simulink model "gm_sampleModel1976_sub"  (R2023a)
settings: Solver=VariableStepAuto  StartTime=0.0  StopTime=10.0  RelTol=1e-3
libraries: simulink x1, hdlsllib x1
settings Model: Creator=user1  LastModifiedBy=user1
settings OptimizationCC: BlockReduction=off  ConditionallyExecuteInputs=off
settings DebuggingCC: InheritedTsInSrcMsg=none

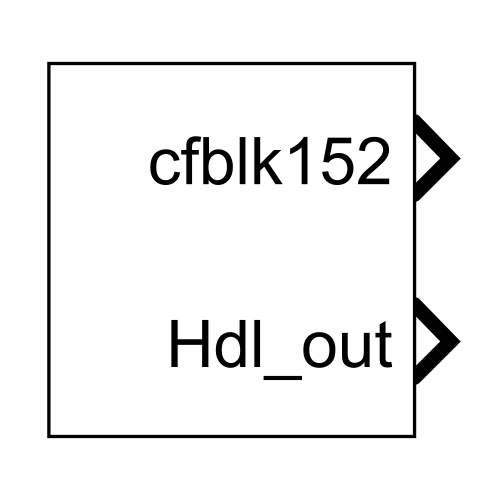
[thumbnail: Simulink's stored preview of the top-level diagram]
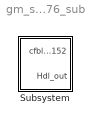
== system gm_sampleModel1976_sub ==
  Subsystem : Subsystem

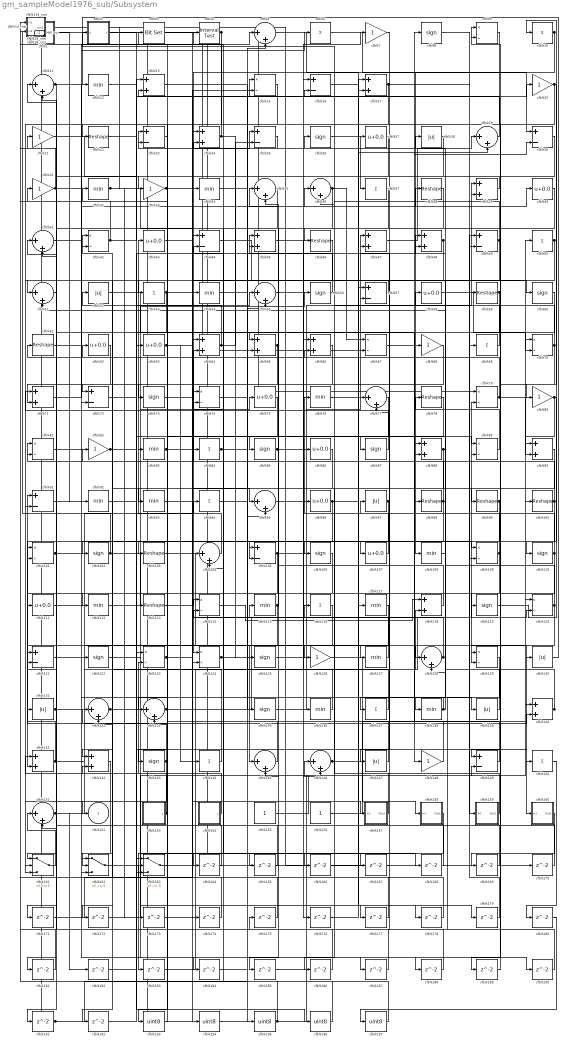
== system gm_sampleModel1976_sub/Subsystem ==
  cfblk1 : Subsystem  mask(Compare To Constant){relop=<=, const=double(3), OutDataTypeStr=uint8, ZeroCross=on}
      mask prompts: relop "Simulink:masks:Operator_MP"; const "Simulink:masks:ConstantValue_MP"; OutDataTypeStr "Simulink:masks:OutputDataType_MP"; ZeroCross "Simulink:masks:EnableZerocrossingDetection_MP"
      mask help: Simulink:masks:CompareToConstant_MD
      mask init:
      | OutDataTypeStr = 'uint8';
      | ZeroCross = 'on';
      | blkName = 'sampleModel1976_sub/Subsystem/cfblk1';
      | const = double(3);
      | const_str = '3.0';
      | const_val = double(3);
      | relop = '<=';
      | setValue = 'fixdt(0, 8)';
      | str = '<= 3';
      mask TypeOptions relop: == | ~= | < | <= | >= | >
      mask TypeOptions OutDataTypeStr: Simulink:masks:uint8 | Simulink:masks:boolean
      mask Callback ZeroCross: sl('zeroCrossEnable', gcbh);
      mask Display: disp(str)
  cfblk{6,10,37,50,53,69,84,94,116,137,144,150} (12 alike) : Sum  Inputs=+  OutDataTypeStr=uint8
  cfblk{22,38,46,59,61,78,98..100,103,113} (11 alike) : Reshape
  cfblk{9,15,42,67,70,74,79,81,89,101,109,114,120,123..124,129} (16 alike) : Product  Inputs=*/  OutDataTypeStr=uint8  RndMeth=Zero  SaturateOnIntegerOverflow=on
  cfblk{8,26,56,60,73,85,87,102,106,110,119,122,125,135,143} (15 alike) : Signum
  cfblk{5,11,29,35..36,41,51,55,77,95,104,128,132..133,145..146,151} (17 alike) : Sum  Inputs=|++  OutDataTypeStr=uint8
  cfblk{16,23,25,30,44,49,57,72,91,105,121,149} (12 alike) : Sum  Inputs=+-  OutDataTypeStr=uint8
  cfblk{27,40,43,58,62..63,75,86,96,107,111} (11 alike) : Bias  Bias=0.0  SaturateOnIntegerOverflow=off
  cfblk{12,32,34,54,76,83,92..93,108,112,115,117,127,136,138} (15 alike) : MinMax  OutDataTypeStr=uint8
  cfblk{13,17,24,39,45,47..48,64..66,71,88,90,118,140..142} (17 alike) : Sum  OutDataTypeStr=uint8
  cfblk{7,20..21,31,33,68,80,82,126,148} (10 alike) : Gain  OutDataTypeStr=uint8
  cfblk{28,52,97,130..131,139,147} (7 alike) : Abs  OutDataTypeStr=uint8  SaturateOnIntegerOverflow=off
  cfblk134_inst : Subsystem
  cfblk14_inst : Subsystem
  cfblk153 : Subsystem  mask(Counter Limited){uplimit=double(7), tsamp=double(-1)}
      mask prompts: uplimit "Simulink:masks:UpperLimit_MP"; tsamp "Simulink:masks:SampleTime_MP"
      mask help: Simulink:masks:CounterLimited_MD
      mask init:
      | nbits = double(8);
      | tsamp = double(-1);
      | uplimit = double(7);
  cfblk154 : Subsystem  mask(Counter Limited){uplimit=double(7), tsamp=double(-1)}
      mask prompts: uplimit "Simulink:masks:UpperLimit_MP"; tsamp "Simulink:masks:SampleTime_MP"
      mask help: Simulink:masks:CounterLimited_MD
      mask init:
      | nbits = double(8);
      | tsamp = double(-1);
      | uplimit = double(7);
  cfblk155 : Constant  OutDataTypeStr=uint8  SampleTime=-1
  cfblk156 : Constant  OutDataTypeStr=uint8  SampleTime=-1
  cfblk157 : Subsystem
  cfblk158 : Subsystem
  cfblk159 : Subsystem
  cfblk160 : Subsystem
  cfblk161 : Switch  OutDataTypeStr=uint8  SaturateOnIntegerOverflow=off  InputSameDT=off
  cfblk162 : Switch  OutDataTypeStr=uint8  SaturateOnIntegerOverflow=off  InputSameDT=off
  cfblk163 : Switch  OutDataTypeStr=uint8  SaturateOnIntegerOverflow=off  InputSameDT=off
  cfblk{164..192} (29 alike) : Delay  SampleTime=1
  cfblk18_inst : Subsystem
  cfblk{193..197} (5 alike) : DataTypeConversion  OutDataTypeStr=uint8  SaturateOnIntegerOverflow=off  RndMeth=Floor
  cfblk19_inst : Subsystem
  cfblk2 : Subsystem  mask(Detect Rise Nonnegative){vinit=double(0), InputProcessing=Elements as channels (sample based), OutDataTypeStr=uint8}
      mask prompts: vinit "Simulink:masks:InitialCondition_MP"; InputProcessing "Simulink:masks:InputProcessing_MP"; OutDataTypeStr "Simulink:masks:OutputDataType_MP"
      mask help: Simulink:masks:DetectRiseNonnegative_MD
      mask init:
      | InputProcessing = 'Elements as channels (sample based)';
      | OutDataTypeStr = 'uint8';
      | vinit = double(0);
      mask TypeOptions InputProcessing: Simulink:masks:ColumnsAsChannelsFrameBased | Simulink:masks:ElementsAsChannelsSampleBased
      mask TypeOptions OutDataTypeStr: Simulink:masks:uint8 | Simulink:masks:boolean
      mask Display: fprintf('U >= 0\n&  NOT\nU/z >= 0')
  cfblk3 : simulink/Logic and Bit Operations/Bit Set  iBit=0
      settings: LibrarySourceBlock=|
      | hdlsllib/Logic and Bit
      | Operations/Bit Set
  cfblk4 : hdlsllib/Logic and Bit Operations/Interval Test  IntervalClosedRight=on  uplimit=0.5  IntervalClosedLeft=on  lowlimit=-0.5  OutDataTypeStr=uint8
  cfblk152 : Outport  OutDataTypeStr=uint8  SampleTime=1  VectorParamsAs1DForOutWhenUnconnected=off
  Hdl_out : Outport  Port=2  OutDataTypeStr=uint8  SampleTime=1
  wires:
  cfblk1/1(y) -> cfblk92/1
  cfblk10/1 -> cfblk124/1, cfblk108/1
  cfblk100/1 -> cfblk64/2, cfblk141/2, cfblk79/2
  cfblk101/1 -> cfblk118/2, cfblk94/1, cfblk54/1
  cfblk102/1 -> cfblk56/1, cfblk19_inst/2(in2), cfblk177/1
  cfblk103/1 -> cfblk160/1(In1)
  cfblk104/1 -> cfblk43/1
  cfblk105/1 -> cfblk47/1, cfblk39/1, cfblk151/2
  cfblk106/1 -> cfblk115/1
  cfblk107/1 -> cfblk97/1
  cfblk108/1 -> cfblk138/1
  cfblk109/1 -> cfblk129/2, cfblk76/1
  cfblk11/1 -> cfblk122/1, cfblk191/1
  cfblk110/1 -> cfblk161/1, cfblk9/1
  cfblk111/1 -> cfblk145/1
  cfblk112/1 -> cfblk75/1
  cfblk113/1 -> cfblk114/1
  cfblk114/1 -> cfblk118/1
  cfblk115/1 -> cfblk35/2, cfblk124/2
  cfblk116/1 -> cfblk181/1
  cfblk117/1 -> cfblk162/2
  cfblk118/1 -> cfblk35/1
  cfblk119/1 -> cfblk10/1
  cfblk12/1 -> cfblk113/1
  cfblk120/1 -> cfblk58/1, cfblk149/1
  cfblk121/1 -> cfblk188/1
  cfblk122/1 -> cfblk190/1
  cfblk123/1 -> cfblk25/1, cfblk120/2
  cfblk124/1 -> cfblk130/1, cfblk89/2
  cfblk125/1 -> cfblk57/2
  cfblk126/1 -> cfblk158/1(In1)
  cfblk127/1 -> cfblk66/2
  cfblk128/1 -> cfblk114/2, cfblk116/1
  cfblk129/1 -> cfblk175/1
  cfblk13/1 -> cfblk55/2
  cfblk130/1 -> cfblk12/1
  cfblk131/1 -> cfblk88/2, cfblk66/1, cfblk16/1
  cfblk132/1 -> cfblk42/1, cfblk168/1
  cfblk133/1 -> cfblk49/2, cfblk68/1
  cfblk134_inst/1(out1) -> cfblk79/1, cfblk170/1
  cfblk135/1 -> cfblk17/2
  cfblk136/1 -> cfblk44/2
  cfblk137/1 -> cfblk74/2
  cfblk138/1 -> cfblk28/1, cfblk137/1
  cfblk139/1 -> cfblk23/1
  cfblk14_inst/1(out1) -> cfblk195/1
  cfblk140/1 -> cfblk62/1, cfblk51/2
  cfblk141/1 -> cfblk91/1, cfblk86/1, cfblk140/2
  cfblk142/1 -> cfblk162/3
  cfblk143/1 -> cfblk23/2, cfblk161/2, cfblk131/1
  cfblk144/1 -> cfblk82/1
  cfblk145/1 -> cfblk61/1
  cfblk146/1 -> cfblk140/1, cfblk120/1
  cfblk147/1 -> cfblk32/1
  cfblk148/1 -> cfblk31/1
  cfblk149/1 -> cfblk81/1
  cfblk15/1 -> cfblk103/1
  cfblk150/1 -> cfblk180/1
  cfblk151/1 -> cfblk8/1, cfblk182/1, cfblk50/1
  cfblk153/1(y) -> cfblk142/2, cfblk141/1, cfblk123/2
  cfblk154/1(y) -> cfblk121/2
  cfblk155/1 -> cfblk70/1
  cfblk156/1 -> cfblk98/1
  cfblk157/1(Out1) -> cfblk2/1(U)
  cfblk158/1(Out1) -> cfblk183/1
  cfblk159/1(Out1) -> cfblk83/1
  cfblk16/1 -> cfblk117/1
  cfblk160/1(Out1) -> cfblk169/1
  cfblk161/1 -> cfblk151/1
  cfblk162/1 -> cfblk167/1
  cfblk163/1 -> cfblk24/1
  cfblk164/1 -> cfblk41/1
  cfblk165/1 -> cfblk64/1
  cfblk166/1 -> cfblk29/2
  cfblk167/1 -> cfblk1/1(u)
  cfblk168/1 -> cfblk13/2
  cfblk169/1 -> cfblk17/1
  cfblk17/1 -> cfblk133/2, cfblk101/2, cfblk159/1(In1)
  cfblk170/1 -> cfblk44/1
  cfblk171/1 -> cfblk74/1
  cfblk172/1 -> cfblk149/2
  cfblk173/1 -> cfblk5/2
  cfblk174/1 -> cfblk42/2
  cfblk175/1 -> cfblk163/2
  cfblk176/1 -> cfblk77/1
  cfblk177/1 -> cfblk132/1
  cfblk178/1 -> cfblk134_inst/1(in1)
  cfblk179/1 -> cfblk49/1
  cfblk18_inst/1(out1) -> cfblk67/2
  cfblk180/1 -> cfblk197/1
  cfblk181/1 -> cfblk19_inst/1(in1)
  cfblk182/1 -> cfblk55/1
  cfblk183/1 -> cfblk146/1
  cfblk184/1 -> cfblk65/2
  cfblk185/1 -> cfblk57/1
  cfblk186/1 -> cfblk81/2
  cfblk187/1 -> cfblk163/1
  cfblk188/1 -> cfblk47/2
  cfblk189/1 -> cfblk9/2
  cfblk19_inst/1(out1) -> cfblk34/1
  cfblk190/1 -> cfblk11/2
  cfblk191/1 -> cfblk95/2, Hdl_out/1
  cfblk192/1 -> cfblk63/1
  cfblk193/1 -> cfblk3/1
  cfblk194/1 -> cfblk119/1
  cfblk195/1 -> cfblk104/2, cfblk100/1
  cfblk196/1 -> cfblk14_inst/1(in1)
  cfblk197/1 -> cfblk14_inst/2(in2)
  cfblk2/1(Y) -> cfblk88/1
  cfblk20/1 -> cfblk80/1, cfblk129/1
  cfblk21/1 -> cfblk123/1
  cfblk22/1 -> cfblk65/1
  cfblk23/1 -> cfblk73/1
  cfblk24/1 -> cfblk18_inst/1(in1), cfblk125/1
  cfblk25/1 -> cfblk24/2
  cfblk26/1 -> cfblk37/1
  cfblk27/1 -> cfblk41/2
  cfblk28/1 -> cfblk121/1
  cfblk29/1 -> cfblk13/1
  cfblk3/1 -> cfblk194/1
  cfblk30/1 -> cfblk99/1
  cfblk31/1 -> cfblk5/1, cfblk18_inst/2(in2), cfblk106/1, cfblk105/2
  cfblk32/1 -> cfblk174/1, cfblk173/1
  cfblk33/1 -> cfblk87/1, cfblk187/1
  cfblk34/1 -> cfblk89/1
  cfblk35/1 -> cfblk104/1
  cfblk36/1 -> cfblk145/2, cfblk67/1
  cfblk37/1 -> cfblk101/1
  cfblk38/1 -> cfblk51/1
  cfblk39/1 -> cfblk33/1
  cfblk4/1 -> cfblk91/2, cfblk171/1
  cfblk40/1 -> cfblk46/1
  cfblk41/1 -> cfblk40/1
  cfblk42/1 -> cfblk134_inst/2(in2), cfblk15/1
  cfblk43/1 -> cfblk60/1
  cfblk44/1 -> cfblk146/2
  cfblk45/1 -> cfblk176/1
  cfblk46/1 -> cfblk84/1
  cfblk47/1 -> cfblk29/1
  cfblk48/1 -> cfblk162/1, cfblk161/3, cfblk132/2
  cfblk49/1 -> cfblk85/1, cfblk16/2
  cfblk5/1 -> cfblk27/1
  cfblk50/1 -> cfblk128/2, cfblk185/1
  cfblk51/1 -> cfblk11/1
  cfblk52/1 -> cfblk148/1
  cfblk53/1 -> cfblk95/1, cfblk71/2
  cfblk54/1 -> cfblk36/1
  cfblk55/1 -> cfblk136/1
  cfblk56/1 -> cfblk45/1
  cfblk57/1 -> cfblk53/1
  cfblk58/1 -> cfblk70/2
  cfblk59/1 -> cfblk147/1, cfblk172/1
  cfblk6/1 -> cfblk30/1
  cfblk60/1 -> cfblk72/1
  cfblk61/1 -> cfblk184/1
  cfblk62/1 -> cfblk111/1
  cfblk63/1 -> cfblk15/2, cfblk144/1
  cfblk64/1 -> cfblk52/1, cfblk25/2
  cfblk65/1 -> cfblk163/3, cfblk112/1
  cfblk66/1 -> cfblk105/1
  cfblk67/1 -> cfblk30/2
  cfblk68/1 -> cfblk72/2
  cfblk69/1 -> cfblk26/1
  cfblk7/1 -> cfblk127/1
  cfblk70/1 -> cfblk36/2, cfblk189/1
  cfblk71/1 -> cfblk6/1
  cfblk72/1 -> cfblk150/1
  cfblk73/1 -> cfblk109/1
  cfblk74/1 -> cfblk135/1
  cfblk75/1 -> cfblk164/1
  cfblk76/1 -> cfblk59/1
  cfblk77/1 -> cfblk193/1
  cfblk78/1 -> cfblk133/1
  cfblk79/1 -> cfblk90/1, cfblk4/1
  cfblk8/1 -> cfblk69/1
  cfblk80/1 -> cfblk90/2, cfblk110/1
  cfblk81/1 -> cfblk107/1
  cfblk82/1 -> cfblk45/2, cfblk192/1
  cfblk83/1 -> cfblk39/2, cfblk157/1(In1)
  cfblk84/1 -> cfblk38/1, cfblk20/1
  cfblk85/1 -> cfblk96/1, cfblk178/1, cfblk109/2
  cfblk86/1 -> cfblk93/1
  cfblk87/1 -> cfblk71/1
  cfblk88/1 -> cfblk48/1, cfblk186/1
  cfblk89/1 -> cfblk78/1
  cfblk9/1 -> cfblk22/1
  cfblk90/1 -> cfblk102/1
  cfblk91/1 -> cfblk139/1
  cfblk92/1 -> cfblk196/1
  cfblk93/1 -> cfblk48/2
  cfblk94/1 -> cfblk126/1
  cfblk95/1 -> cfblk7/1
  cfblk96/1 -> cfblk142/1, cfblk128/1, cfblk179/1
  cfblk97/1 -> cfblk77/2, cfblk166/1
  cfblk98/1 -> cfblk143/1, cfblk21/1
  cfblk99/1 -> cfblk165/1, cfblk152/1

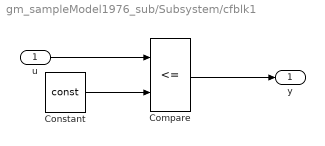
== system gm_sampleModel1976_sub/Subsystem/cfblk1 ==
  u : Inport  OutDataTypeStr=uint8  SampleTime=1
  Compare : RelationalOperator  Operator=<=  OutDataTypeStr=fixdt(0, 8)
  Constant : Constant  DisableCoverage=on  Value=const  OutDataTypeStr=Inherit: Inherit via back propagation  SampleTime=-1
  y : Outport  SampleTime=1
  wires:
  u/1 -> Compare/1
  Compare/1 -> y/1
  Constant/1 -> Compare/2

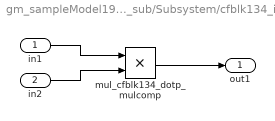
== system gm_sampleModel1976_sub/Subsystem/cfblk134_inst ==
  in1 : Inport  OutDataTypeStr=uint8  SampleTime=1
  in2 : Inport  Port=2  OutDataTypeStr=uint8  SampleTime=1
  mul_cfblk134_dotp_mulcomp : Product  Inputs=**  OutDataTypeStr=uint8  SampleTime=1
  out1 : Outport  OutDataTypeStr=uint8  SampleTime=1
  wires:
  in1/1 -> mul_cfblk134_dotp_mulcomp/1
  in2/1 -> mul_cfblk134_dotp_mulcomp/2
  mul_cfblk134_dotp_mulcomp/1 -> out1/1

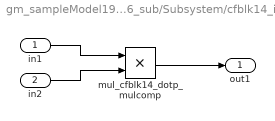
== system gm_sampleModel1976_sub/Subsystem/cfblk14_inst ==
  in1 : Inport  OutDataTypeStr=uint8  SampleTime=1
  in2 : Inport  Port=2  OutDataTypeStr=uint8  SampleTime=1
  mul_cfblk14_dotp_mulcomp : Product  Inputs=**  OutDataTypeStr=uint8  SampleTime=1
  out1 : Outport  OutDataTypeStr=uint8  SampleTime=1
  wires:
  in1/1 -> mul_cfblk14_dotp_mulcomp/1
  in2/1 -> mul_cfblk14_dotp_mulcomp/2
  mul_cfblk14_dotp_mulcomp/1 -> out1/1

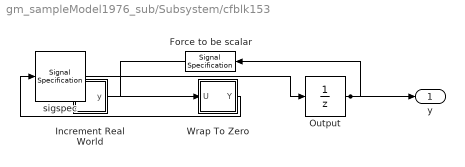
== system gm_sampleModel1976_sub/Subsystem/cfblk153 ==
  Force to be scalar : SignalSpecification  DisableCoverage=on  Dimensions=1
  Increment Real World : Subsystem  mask(Real World Value Increment){}
      mask help: Simulink:masks:RealWorldValueIncrement_MD
      mask Display: disp('V++')
  Output : UnitDelay  InitialCondition=0.0  SampleTime=tsamp  HasFrameUpgradeWarning=on
  Wrap To Zero : Subsystem  mask(Wrap To Zero){Threshold=double(7)}
      mask prompts: Threshold "Simulink:masks:Threshold_MP"
      mask help: Simulink:masks:WrapToZero_MD
  sigspec : SignalSpecification  OutDataTypeStr=uint8  Dimensions=1
  y : Outport  SampleTime=1
  wires:
  Force to be scalar/1 -> Increment Real World/1(u)
  Increment Real World/1(y) -> Wrap To Zero/1(U)
  Output/1 -> Force to be scalar/1, y/1
  Wrap To Zero/1(Y) -> sigspec/1
  sigspec/1 -> Output/1

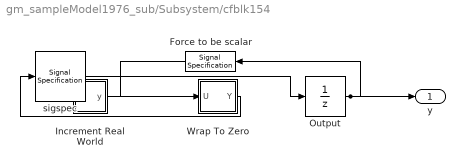
== system gm_sampleModel1976_sub/Subsystem/cfblk154 ==
  Force to be scalar : SignalSpecification  DisableCoverage=on  Dimensions=1
  Increment Real World : Subsystem  mask(Real World Value Increment){}
      mask help: Simulink:masks:RealWorldValueIncrement_MD
      mask Display: disp('V++')
  Output : UnitDelay  InitialCondition=0.0  SampleTime=tsamp  HasFrameUpgradeWarning=on
  Wrap To Zero : Subsystem  mask(Wrap To Zero){Threshold=double(7)}
      mask prompts: Threshold "Simulink:masks:Threshold_MP"
      mask help: Simulink:masks:WrapToZero_MD
  sigspec : SignalSpecification  OutDataTypeStr=uint8  Dimensions=1
  y : Outport  SampleTime=1
  wires:
  Force to be scalar/1 -> Increment Real World/1(u)
  Increment Real World/1(y) -> Wrap To Zero/1(U)
  Output/1 -> Force to be scalar/1, y/1
  Wrap To Zero/1(Y) -> sigspec/1
  sigspec/1 -> Output/1

== system gm_sampleModel1976_sub/Subsystem/cfblk157 ==
  In1 : Inport  OutDataTypeStr=uint8  PortDimensions=1  SampleTime=1
  Out1 : Outport  SampleTime=1
  wires:
  In1/1 -> Out1/1

== system gm_sampleModel1976_sub/Subsystem/cfblk158 ==
  In1 : Inport  OutDataTypeStr=uint8  PortDimensions=1  SampleTime=1
  Out1 : Outport  SampleTime=1
  wires:
  In1/1 -> Out1/1

== system gm_sampleModel1976_sub/Subsystem/cfblk159 ==
  In1 : Inport  OutDataTypeStr=uint8  PortDimensions=1  SampleTime=1
  Out1 : Outport  SampleTime=1
  wires:
  In1/1 -> Out1/1

== system gm_sampleModel1976_sub/Subsystem/cfblk160 ==
  In1 : Inport  OutDataTypeStr=uint8  PortDimensions=1  SampleTime=1
  Out1 : Outport  SampleTime=1
  wires:
  In1/1 -> Out1/1

== system gm_sampleModel1976_sub/Subsystem/cfblk18_inst ==
  in1 : Inport  OutDataTypeStr=uint8  SampleTime=1
  in2 : Inport  Port=2  OutDataTypeStr=uint8  SampleTime=1
  mul_cfblk18_dotp_mulcomp : Product  Inputs=**  OutDataTypeStr=uint8  SampleTime=1
  out1 : Outport  OutDataTypeStr=uint8  SampleTime=1
  wires:
  in1/1 -> mul_cfblk18_dotp_mulcomp/1
  in2/1 -> mul_cfblk18_dotp_mulcomp/2
  mul_cfblk18_dotp_mulcomp/1 -> out1/1

== system gm_sampleModel1976_sub/Subsystem/cfblk19_inst ==
  in1 : Inport  OutDataTypeStr=uint8  SampleTime=1
  in2 : Inport  Port=2  OutDataTypeStr=uint8  SampleTime=1
  mul_cfblk19_dotp_mulcomp : Product  Inputs=**  OutDataTypeStr=uint8  SampleTime=1
  out1 : Outport  OutDataTypeStr=uint8  SampleTime=1
  wires:
  in1/1 -> mul_cfblk19_dotp_mulcomp/1
  in2/1 -> mul_cfblk19_dotp_mulcomp/2
  mul_cfblk19_dotp_mulcomp/1 -> out1/1

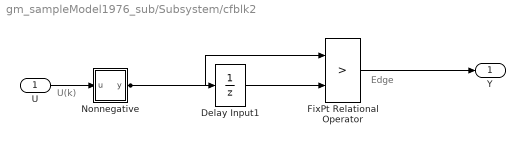
== system gm_sampleModel1976_sub/Subsystem/cfblk2 ==
  note: U(k)
  note: Edge
  U : Inport  OutDataTypeStr=uint8  SampleTime=1
  Delay Input1 : UnitDelay  Description=Store in Global RAM  DisableCoverage=on  InitialCondition=vinit  SampleTime=-1  HasFrameUpgradeWarning=on
  FixPt Relational Operator : RelationalOperator  Operator=>  OutDataTypeStr=fixdt(0, 8)  ZeroCross=off  InputSameDT=off
  Nonnegative : Subsystem  mask(Compare To Zero){relop=>=, OutDataTypeStr=boolean, ZeroCross=off}
      mask prompts: relop "Simulink:masks:Operator_MP"; OutDataTypeStr "Simulink:masks:OutputDataType_MP"; ZeroCross "Simulink:masks:EnableZerocrossingDetection_MP"
      mask help: Simulink:masks:CompareToZero_MD
      mask init:
      | OutDataTypeStr = 'boolean';
      | ZeroCross = 'off';
      | blkName = 'sampleModel1976_sub/Subsystem/cfblk2/Nonnegative';
      | relop = '>=';
      | setValue = 'boolean';
      mask TypeOptions relop: == | ~= | < | <= | >= | >
      mask TypeOptions OutDataTypeStr: Simulink:masks:uint8 | Simulink:masks:boolean
      mask Callback ZeroCross: sl('zeroCrossEnable', gcbh);
      mask Display: disp([relop,' 0'])
  Y : Outport  SampleTime=1
  wires:
  U/1 -> Nonnegative/1(u)
  Delay Input1/1 -> FixPt Relational Operator/2
  FixPt Relational Operator/1 -> Y/1
  Nonnegative/1(y) -> FixPt Relational Operator/1, Delay Input1/1

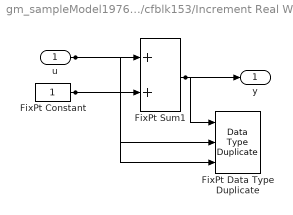
== system gm_sampleModel1976_sub/Subsystem/cfblk153/Increment Real World ==
  u : Inport  OutDataTypeStr=uint8  SampleTime=1
  FixPt Constant : Constant  DisableCoverage=on  OutDataTypeStr=Inherit: Inherit via back propagation  SampleTime=-1
  FixPt Data Type Duplicate : DataTypeDuplicate  DisableCoverage=on  NumInputPorts=3
  FixPt Sum1 : Sum  InputSameDT=on  OutDataTypeStr=Inherit: Inherit via back propagation  LockScale=on
  y : Outport  SampleTime=1
  wires:
  u/1 -> FixPt Sum1/1, FixPt Data Type Duplicate/2
  FixPt Constant/1 -> FixPt Sum1/2, FixPt Data Type Duplicate/3
  FixPt Sum1/1 -> FixPt Data Type Duplicate/1, y/1

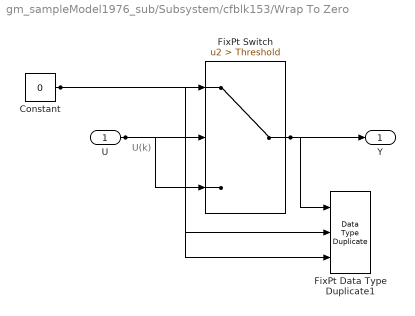
== system gm_sampleModel1976_sub/Subsystem/cfblk153/Wrap To Zero ==
  note: U(k)
  U : Inport  OutDataTypeStr=uint8  SampleTime=1
  Constant : Constant  DisableCoverage=on  Value=0  OutDataTypeStr=Inherit: Inherit via back propagation  SampleTime=-1
  FixPt Data Type Duplicate1 : DataTypeDuplicate  DisableCoverage=on  NumInputPorts=3
  FixPt Switch : Switch  Criteria=u2 > Threshold  Threshold=Threshold  OutDataTypeStr=Inherit: Inherit via back propagation  ZeroCross=off  SaturateOnIntegerOverflow=off  InputSameDT=off
  Y : Outport  SampleTime=1
  wires:
  U/1 -> FixPt Switch/3, FixPt Switch/2, FixPt Data Type Duplicate1/2
  Constant/1 -> FixPt Switch/1, FixPt Data Type Duplicate1/3
  FixPt Switch/1 -> FixPt Data Type Duplicate1/1, Y/1

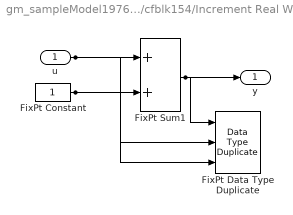
== system gm_sampleModel1976_sub/Subsystem/cfblk154/Increment Real World ==
  u : Inport  OutDataTypeStr=uint8  SampleTime=1
  FixPt Constant : Constant  DisableCoverage=on  OutDataTypeStr=Inherit: Inherit via back propagation  SampleTime=-1
  FixPt Data Type Duplicate : DataTypeDuplicate  DisableCoverage=on  NumInputPorts=3
  FixPt Sum1 : Sum  InputSameDT=on  OutDataTypeStr=Inherit: Inherit via back propagation  LockScale=on
  y : Outport  SampleTime=1
  wires:
  u/1 -> FixPt Sum1/1, FixPt Data Type Duplicate/2
  FixPt Constant/1 -> FixPt Sum1/2, FixPt Data Type Duplicate/3
  FixPt Sum1/1 -> FixPt Data Type Duplicate/1, y/1

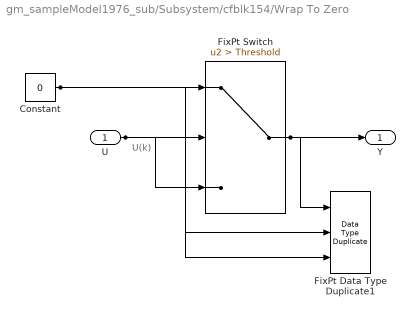
== system gm_sampleModel1976_sub/Subsystem/cfblk154/Wrap To Zero ==
  note: U(k)
  U : Inport  OutDataTypeStr=uint8  SampleTime=1
  Constant : Constant  DisableCoverage=on  Value=0  OutDataTypeStr=Inherit: Inherit via back propagation  SampleTime=-1
  FixPt Data Type Duplicate1 : DataTypeDuplicate  DisableCoverage=on  NumInputPorts=3
  FixPt Switch : Switch  Criteria=u2 > Threshold  Threshold=Threshold  OutDataTypeStr=Inherit: Inherit via back propagation  ZeroCross=off  SaturateOnIntegerOverflow=off  InputSameDT=off
  Y : Outport  SampleTime=1
  wires:
  U/1 -> FixPt Switch/3, FixPt Switch/2, FixPt Data Type Duplicate1/2
  Constant/1 -> FixPt Switch/1, FixPt Data Type Duplicate1/3
  FixPt Switch/1 -> FixPt Data Type Duplicate1/1, Y/1

== system gm_sampleModel1976_sub/Subsystem/cfblk2/Nonnegative ==
  u : Inport  OutDataTypeStr=uint8  SampleTime=1
  Compare : RelationalOperator  OutDataTypeStr=boolean  ZeroCross=off
  Constant : Constant  DisableCoverage=on  Value=0  OutDataTypeStr=Inherit: Inherit via back propagation  SampleTime=-1  PreserveConstantTs=on
  y : Outport  SampleTime=1
  wires:
  u/1 -> Compare/1
  Compare/1 -> y/1
  Constant/1 -> Compare/2
